simulink model "fig4_22_simulink"  (R2021b)
settings: Solver=ode3  StartTime=0.0  StopTime=1000  FixedStep=1e-03  RelTol=1e-3  EnableMultiTasking=on
settings Model: Creator=Nima  LastModifiedBy=One Informatic
settings SolverCC: AlgebraicLoopSolver=TrustRegion
settings DataIOCC: LimitDataPoints=on  SaveFormat=Array  ReturnWorkspaceOutputs=off
settings OptimizationCC: LifeSpan=inf
settings DebuggingCC: SolverPrmCheckMsg=warning  SFUnexpectedBacktrackingDiag=warning  SFNoUnconditionalDefaultTransitionDiag=warning  SFExecutionAtInitializationDiag=none  SFMachineParentedDataDiag=warning  ArithmeticOperatorsInVariantConditions=warning
settings HardwareCC: ProdBitPerPointer=32  ProdBitPerSizeT=32  ProdBitPerPtrDiffT=32  ProdLargestAtomicFloat=None  ProdIntDivRoundTo=Undefined  ProdEndianess=Unspecified  ProdWordSize=32  ProdHWDeviceType=32-bit Generic
settings ModelReferenceCC: PropagateSignalLabelsOutOfModel=off
settings SFSimCC: SimUseLocalCustomCode=off  CustomCodeUndefinedFunction=UseInterfaceOnly
settings RTWCC: RTWUseLocalCustomCode=off
settings CodeAppCC: StateflowObjectComments=on
settings GRTTargetCC: TargetLangStandard=C89/C90 (ANSI)
settings ConfigComp: CovMetricSettings=dw  CovSaveCumulativeToWorkspaceVar=on  CovSaveSingleToWorkspaceVar=on  CovExternalEMLEnable=off  CovSFcnEnable=off

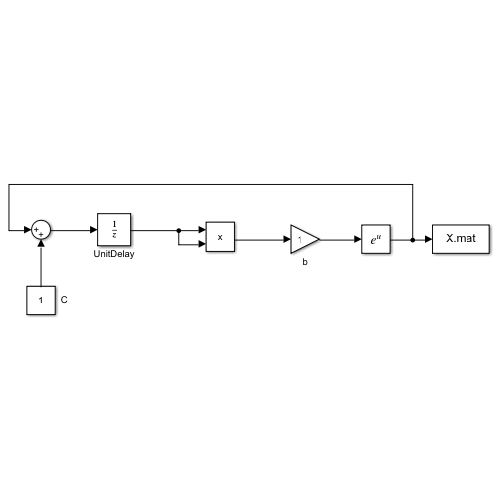
[thumbnail: Simulink's stored preview of the top-level diagram]
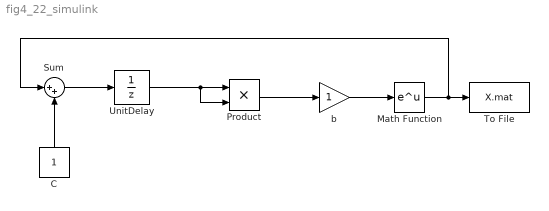
== system fig4_22_simulink ==
  C : Constant
  Math Function : Math  SaturateOnIntegerOverflow=on
  Product : Product
  Sum : Sum  Inputs=|++
  To File : ToFile  Filename=X.mat  MatrixName=X  SampleTime=0.0001
  UnitDelay : UnitDelay  SampleTime=-1  HasFrameUpgradeWarning=on
  b : Gain
  wires:
  C/1 -> Sum/2
  Sum/1 -> UnitDelay/1
  UnitDelay/1 -> Product/2, Product/1
  Product/1 -> b/1
  b/1 -> Math Function/1
  Math Function/1 -> To File/1, Sum/1
